simulink library "csc_rigid_body_dynamics_lib"  (R2014b)
settings: Solver=ode45  SolverMode=SingleTasking  StartTime=0.0  StopTime=10.0  RelTol=1e-3
undefined symbols (not defined in the file): ini_landed_flag, ini_thrust_to_weight_takeoff_limit
libraries: simulink x2, util_frame_rotation_lib x2, util_info_lib x1, csc_eom_six_dof_integration_lib x1, csc_kin_kinematic_propagation_lib x1, csu_ini_initial_conditions_lib x1, csu_lan_landed_state_determination_lib x1, util_common_lib x1
settings Model: ExtModeAutoUpdateStatusClock=off  Creator=daniloviazzo  LastModifiedBy=jimkaidy

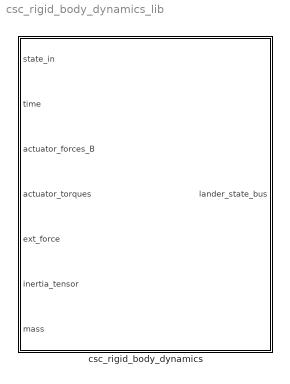
== system csc_rigid_body_dynamics_lib ==
  csc_rigid_body_dynamics : Subsystem

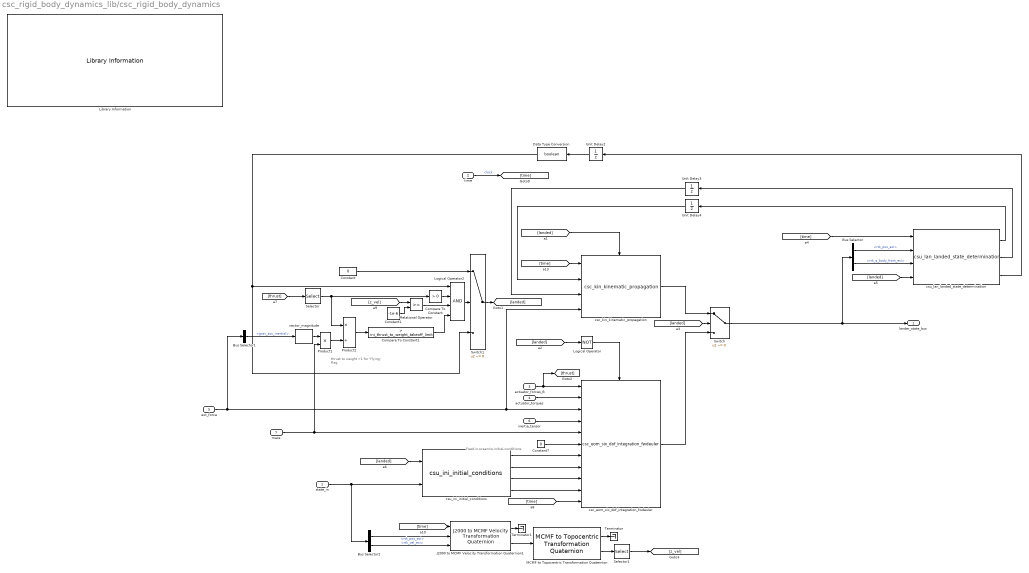
== system csc_rigid_body_dynamics_lib/csc_rigid_body_dynamics ==
  note: Feed in sceanrio initial conditions
  note: thrust to weight >1 for
      | 'flying' flag
  state_in : Inport
  time : Inport  Port=2
  actuator_forces_B : Inport  Port=3
  actuator_torques : Inport  Port=4
  ext_force : Inport  Port=5
  inertia_tensor : Inport  Port=6
  mass : Inport  Port=7
  Bus Selector : BusSelector  OutputSignals=rtk_pos_eci,rrk_q_body_from_eci
  Bus Selector1 : BusSelector  OutputSignals=grav_acc_inertial
  Bus Selector2 : BusSelector  OutputSignals=rtk_pos_eci,rtk_vel_eci
  Compare To Constant : simulink/Logic and Bit Operations/Compare To Constant  relop=>  const=0  OutDataTypeStr=boolean
  Compare To Constant1 : simulink/Logic and Bit Operations/Compare To Constant  relop=>  const=ini_thrust_to_weight_takeoff_limit  OutDataTypeStr=boolean
  Constant : Constant  Value=0  OutDataTypeStr=boolean
  Constant1 : Constant  Value=-1e-6
  Constant7 : Constant  Value=0
  Data Type Conversion : DataTypeConversion  OutDataTypeStr=boolean
  J2000 to MCMF Velocity Transformation Quaternion1 : util_frame_rotation_lib/J2000 to MCMF Velocity Transformation Quaternion  SystemSampleTime=-1
  Library Information : util_info_lib/Library Information  owner='escrane'
  Logical Operator : Logic  Operator=NOT  AllPortsSameDT=off  OutDataTypeStr=boolean
  Logical Operator2 : Logic  Inputs=4  AllPortsSameDT=off  OutDataTypeStr=boolean
  MCMF to Topocentric Transformation Quaternion : util_frame_rotation_lib/MCMF to Topocentric  Transformation Quaternion  SystemSampleTime=-1
  Product1 : Product  RndMeth=Zero
  Product2 : Product  Inputs=*/  RndMeth=Zero
  Relational Operator : RelationalOperator  OutDataTypeStr=boolean
  Selector : Selector  InputPortWidth=3  Indices=3
  Selector1 : Selector  InputPortWidth=3  Indices=3
  Switch : Switch  Criteria=u2 ~= 0
  Switch1 : Switch  Criteria=u2 ~= 0
  Terminator : Terminator
  Terminator1 : Terminator
  Unit Delay2 : UnitDelay  InitialCondition=boolean(ini_landed_flag)  SampleTime=-1
  Unit Delay3 : UnitDelay  InitialCondition=[0 0 0 1]  SampleTime=-1
  Unit Delay4 : UnitDelay  InitialCondition=[0 0 0]  SampleTime=-1
  csc_eom_six_dof_integration_fwdeuler : csc_eom_six_dof_integration_lib/csc_eom_six_dof_integration_fwdeuler
  csc_kin_kinematic_propagation : csc_kin_kinematic_propagation_lib/csc_kin_kinematic_propagation
  csu_ini_initial_conditions : csu_ini_initial_conditions_lib/csu_ini_initial_conditions
  csu_lan_landed_state_determination : csu_lan_landed_state_determination_lib/csu_lan_landed_state_determination
  vector_magnitude : util_common_lib/vector_magnitude  SystemSampleTime=-1
  lander_state_bus : Outport
  wires:
  Bus Selector2/1 -> J2000 to MCMF Velocity Transformation Quaternion1/2  "<rtk_pos_eci>"
  [time] -> J2000 to MCMF Velocity Transformation Quaternion1/1
  J2000 to MCMF Velocity Transformation Quaternion1/1 -> Terminator1/1
  MCMF to Topocentric Transformation Quaternion/1 -> Terminator/1
  J2000 to MCMF Velocity Transformation Quaternion1/2 -> MCMF to Topocentric Transformation Quaternion/1
  Relational Operator/1 -> Logical Operator2/3
  [z_vel] -> Relational Operator/1
  Selector1/1 -> [z_vel]
  MCMF to Topocentric Transformation Quaternion/2 -> Selector1/1
  Bus Selector2/2 -> J2000 to MCMF Velocity Transformation Quaternion1/3  "<rtk_vel_eci>"
  [thrust] -> Selector/1
  Unit Delay4/1 -> csc_kin_kinematic_propagation/2
  Unit Delay3/1 -> csc_kin_kinematic_propagation/3
  state_in/1 -> csu_ini_initial_conditions/2, Bus Selector2/1
  csu_lan_landed_state_determination/2 -> Unit Delay3/1
  csu_lan_landed_state_determination/1 -> Unit Delay4/1
  csc_kin_kinematic_propagation/1 -> Switch/1
  csc_eom_six_dof_integration_fwdeuler/1 -> Switch/3
  Product2/1 -> Compare To Constant1/1
  Compare To Constant1/1 -> Logical Operator2/4
  Compare To Constant/1 -> Logical Operator2/2
  Product1/1 -> Product2/2
  vector_magnitude/1 -> Product1/1
  Selector/1 -> Compare To Constant/1, Product2/1
  Bus Selector1/1 -> vector_magnitude/1  "<grav_acc_inertial>"
  Logical Operator/1 -> csc_eom_six_dof_integration_fwdeuler/Enable
  csu_lan_landed_state_determination/3 -> Unit Delay2/1
  [landed] -> csu_lan_landed_state_determination/4
  Bus Selector/2 -> csu_lan_landed_state_determination/3  "<rrk_q_body_from_eci>"
  Bus Selector/1 -> csu_lan_landed_state_determination/2  "<rtk_pos_eci>"
  [time] -> csu_lan_landed_state_determination/1
  [landed] -> Switch/2
  [landed] -> Logical Operator/1
  [landed] -> csc_kin_kinematic_propagation/Enable
  [time] -> csc_kin_kinematic_propagation/1
  actuator_forces_B/1 -> csc_eom_six_dof_integration_fwdeuler/1, [thrust]
  mass/1 -> Product1/2, csc_eom_six_dof_integration_fwdeuler/5
  Constant7/1 -> csc_eom_six_dof_integration_fwdeuler/6
  inertia_tensor/1 -> csc_eom_six_dof_integration_fwdeuler/4
  csu_ini_initial_conditions/4 -> csc_eom_six_dof_integration_fwdeuler/10
  csu_ini_initial_conditions/3 -> csc_eom_six_dof_integration_fwdeuler/9
  csu_ini_initial_conditions/2 -> csc_eom_six_dof_integration_fwdeuler/8
  csu_ini_initial_conditions/1 -> csc_eom_six_dof_integration_fwdeuler/7
  time/1 -> [time]  "clock"
  Switch/1 -> lander_state_bus/1, Bus Selector/1
  [landed] -> csu_ini_initial_conditions/1
  Logical Operator2/1 -> Switch1/2
  Constant/1 -> Switch1/1
  Unit Delay2/1 -> Data Type Conversion/1
  Data Type Conversion/1 -> Logical Operator2/1, Switch1/3
  [time] -> csc_eom_six_dof_integration_fwdeuler/11
  ext_force/1 -> Bus Selector1/1, csc_eom_six_dof_integration_fwdeuler/3, csc_kin_kinematic_propagation/4
  actuator_torques/1 -> csc_eom_six_dof_integration_fwdeuler/2
  Switch1/1 -> [landed]
  Constant1/1 -> Relational Operator/2
